simulink model "s5"  (Simulink 2.00)
settings: Solver=ode15s  StartTime=0.0  StopTime=35  MaxStep=0.05  RelTol=1e-6  AbsTol=1e-6
values from neighbouring files (symbols this model uses):
  J = 0.8    [M1.M]    (also in M2.M = 2.5; M3A.M = 0.5; M3B.M = 0.5; M4.M = 0.015)
  Laq = 0.018    [M1.M]    (also in M2.M = 0.012; M3A.M; M3B.M; M4.M = 0.01)
  Lse = 0.026    [M4.M]    (also in M5.M = 0.044)
  Ra = 0.24    [M1.M]    (also in M2.M = 0.3; M3A.M = 0.14; M3B.M = 0.14; M4.M = 0.6)
  Rbrake = (Vbrake - kaphibrake*wbrake)/Iabrake - Ra - Rse    [M5.M]
  Rse = 0.1    [M4.M]    (also in M5.M = 0.2)
  SEIP5 = [-27.224 -23.547 -20.624 -18.739 -17.560 -16.617   -15.627 -14.826 -13.977 -13.317 -12.643 -11.969 -11.290  -10.041 -8.886 -7.613 -6.576 -5.647 -4.643 -3.582 -2.521  -1.423 -0.400  0.623  1.721  2.782  3.843  4.847  5.776   6.813  8.086  9.241 10.490 11.169 11.843 12.517 13.177 14.026  14.827 15.817 16.760 17.939 19.824 22.747 26.424 ]    [M5.M]
  SEVP5 = [-160 -155 -150 -145 -140 -135 -130 -125 -120 -115  -110 -105 -100 -90 -80 -70 -60 -50 -40 -30 -20 -10 0  10 20 30 40 50 60 70 80 90 100 105 110 115 120 125 130 135  140 145 150 155 160 ]    [M5.M]
  Trated = Prated/wmrated    (= 8.14145743176)    [M1.M]    (also in M2.M = 47.8105721664; M3A.M; M3B.M; M4.M = 1.10840049653)
  Vbrake = 0    [M3A.M]    (also in M5.M)
  Vmotor = Vrated-2    (= 123)    [M5.M]
  wmo = 2000*(2*pi)/60    (= 209.439510239)    [M1.M]    (also in M4.M = 157.079632679; M5.M = 125.663706144)
settings Model: SaveTime=off  SaveOutput=off  ConsistencyChecking=off

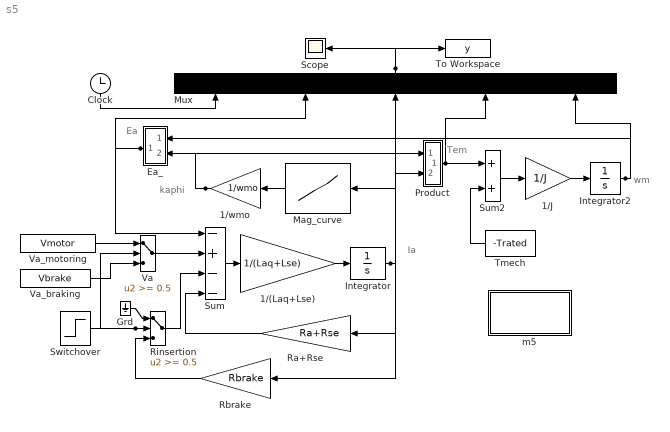
== system s5 ==
  note: Ia
  note: Tem
  note: kaphi
  note: Ea
  note: wm
  1/(Laq+Lse) : Gain  Gain=1/(Laq+Lse)
  1/J : Gain  Gain=1/J
  1/wmo : Gain  Orientation=left  Gain=1/wmo
  Clock : Clock
      settings: Orientation=down  DeleteFcn=simclock BlockIsBeingDestroyed  PostSaveFcn=simclock Save
  Ea_ : Subsystem  Orientation=left
      mask Type: Dot Product
      mask Description:
      | Inner (dot) product.
      | y=sum(u1.*u2)
      mask Help: Computes the inner (dot) product of the inputs: sum(u1.*u2).  The inputs are vectors of the same length. Output is a scalar.
      mask Display: disp('.\n')
  Grd : Ground
  Integrator : Integrator  ExternalReset=none  InitialConditionSource=internal  InitialCondition=0  LimitOutput=off  UpperSaturationLimit=inf  LowerSaturationLimit=-inf  ShowSaturationPort=off  ShowStatePort=off  AbsoluteTolerance=auto
  Integrator2 : Integrator  ExternalReset=none  InitialConditionSource=internal  InitialCondition=0  LimitOutput=off  UpperSaturationLimit=inf  LowerSaturationLimit=-inf  ShowSaturationPort=off  ShowStatePort=off  AbsoluteTolerance=auto
  m5 : Subsystem
      settings: OpenFcn=m5
      mask Type: Masked block of m5.m
      mask Help: Uses m5.m to initialize and plot
      mask Display: disp('Initialize\nand plot')
  Mag_curve : Lookup  Orientation=left  InputValues=SEIP5  OutputValues=SEVP5
  Mux : Mux  Orientation=up  Inputs=5
  Product : Subsystem
      mask Type: Dot Product
      mask Description:
      | Inner (dot) product.
      | y=sum(u1.*u2)
      mask Help: Computes the inner (dot) product of the inputs: sum(u1.*u2).  The inputs are vectors of the same length. Output is a scalar.
      mask Display: disp('.\n')
  Ra+Rse : Gain  Orientation=left  Gain=Ra+Rse
  Rbrake : Gain  Orientation=left  Gain=Rbrake
  Rinsertion : Switch  Threshold=0.5
  Scope : Scope
      settings: TickLabels=on  TimeRange=35  YMin=-150  YMax=150  SaveToWorkspace=off  SaveName=ScopeData  LimitMaxRows=off
  Sum : Sum  Inputs=-+--
  Sum2 : Sum  Inputs=++
  Switchover : Step  Time=8  Before=1  After=0
  Tmech : Constant  Orientation=left  Value=-Trated
  To Workspace : ToWorkspace  VariableName=y  SampleTime=0
      settings: Buffer=20000
  Va : Switch  Threshold=0.5
  Va_braking : Constant  Value=Vbrake
  Va_motoring : Constant  Value=Vmotor
  wires:
  Sum/1 -> 1/(Laq+Lse)/1
  Sum2/1 -> 1/J/1
  1/J/1 -> Integrator2/1
  1/(Laq+Lse)/1 -> Integrator/1
  Clock/1 -> Mux/1
  Mag_curve/1 -> 1/wmo/1
  Tmech/1 -> Sum2/2
  1/wmo/1 -> Product/1(in_1), Ea_/2(in_2)
  Ea_/1(out_1) -> Sum/1, Mux/2
  Integrator/1 -> Ra+Rse/1, Mux/3, Mag_curve/1, Product/2(in_2), Rbrake/1
  Rbrake/1 -> Rinsertion/3
  Ra+Rse/1 -> Sum/4
  Rinsertion/1 -> Sum/3
  Va/1 -> Sum/2
  Va_motoring/1 -> Va/1
  Va_braking/1 -> Va/3
  Switchover/1 -> Rinsertion/2, Va/2
  Integrator2/1 -> Ea_/1(in_1), Mux/5
  Product/1(out_1) -> Sum2/1, Mux/4
  Mux/1 -> To Workspace/1, Scope/1
  Grd/1 -> Rinsertion/1

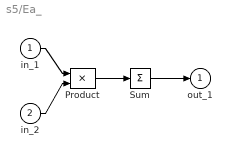
== system s5/Ea_ ==
  in_1 : Inport  Port=1  PortWidth=-1  SampleTime=-1
  in_2 : Inport  Port=2  PortWidth=-1  SampleTime=-1
  Product : Product  Inputs=2
  Sum : Sum  Inputs=+
  out_1 : Outport  Port=1  InitialOutput=0
  wires:
  in_2/1 -> Product/2
  in_1/1 -> Product/1
  Product/1 -> Sum/1
  Sum/1 -> out_1/1

== system s5/m5 ==
  note: Uses m5.m to initialize s5.m
      | and plot results

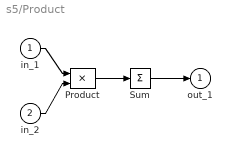
== system s5/Product ==
  in_1 : Inport  Port=1  PortWidth=-1  SampleTime=-1
  in_2 : Inport  Port=2  PortWidth=-1  SampleTime=-1
  Product : Product  Inputs=2
  Sum : Sum  Inputs=+
  out_1 : Outport  Port=1  InitialOutput=0
  wires:
  in_2/1 -> Product/2
  in_1/1 -> Product/1
  Product/1 -> Sum/1
  Sum/1 -> out_1/1
